simulink model "simCRM_Hybrid"  (R2016b)
settings: Solver=ode5  StartTime=0.0  StopTime=SimConfig.EndTime  FixedStep=SimConfig.SampleTime  RelTol=1e-3
undefined symbols (not defined in the file): CRM, WindReconstruction
libraries: lib_Sim_CRM x9, Controllers x1, Lidar_WindReconstruction x1, simulink x1
settings Model: Creator=cava_da  LastModifiedBy=cava_da
settings DataIOCC: Decimation=SimConfig.Logging.DecimationFactor  SaveFormat=StructureWithTime  ReturnWorkspaceOutputs=on
settings OptimizationCC: ExpressionDepthLimit=2147483647  InitFltsAndDblsToZero=on  LifeSpan=inf
settings DebuggingCC: UnderspecifiedInitializationDetection=Classic  MergeDetectMultiDrivingBlocksExec=none  SolverPrmCheckMsg=warning  FcnCallInpInsideContextMsg=warning  StateNameClashWarn=warning  SFUnexpectedBacktrackingDiag=warning  SFNoUnconditionalDefaultTransitionDiag=warning  SFExecutionAtInitializationDiag=none
settings HardwareCC: ProdBitPerPointer=32  ProdBitPerSizeT=32  ProdBitPerPtrDiffT=32  ProdLargestAtomicFloat=None  ProdIntDivRoundTo=Undefined  ProdEndianess=Unspecified  ProdWordSize=32  ProdHWDeviceType=32-bit Generic
settings ModelReferenceCC: PropagateSignalLabelsOutOfModel=off
settings SFSimCC: SimUseLocalCustomCode=on
settings RTWCC: RTWUseLocalCustomCode=on
settings GRTTargetCC: TargetLangStandard=C89/C90 (ANSI)  CombineOutputUpdateFcns=off  GRTInterface=on
settings ConfigComp: CovMetricSettings=dw  CovHtmlReporting=on  CovSaveCumulativeToWorkspaceVar=on  CovSaveSingleToWorkspaceVar=on

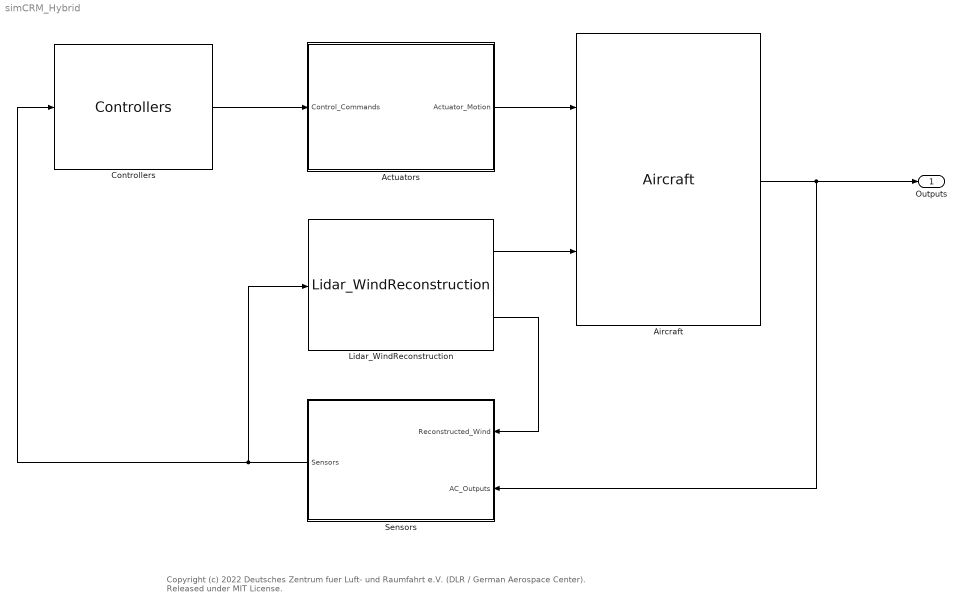
== system simCRM_Hybrid ==
  note: Copyright (c) 2022 Deutsches Zentrum fuer Luft- und Raumfahrt e.V. (DLR / German Aerospace Center). Released under MIT License.
  Actuators : Subsystem
  Aircraft : lib_Sim_CRM/Aircraft  modelName=CRM.Aircraft
  Controllers : Controllers/Controllers  SystemSampleTime=-1
  Lidar_WindReconstruction : Lidar_WindReconstruction/Lidar_WindReconstruction  SystemSampleTime=-1
  Sensors : Subsystem
  Outputs : Outport
  wires:
  Lidar_WindReconstruction/1 -> Aircraft/2
  Aircraft/1 -> Outputs/1, Sensors/2(AC_Outputs)
  Lidar_WindReconstruction/2 -> Sensors/1(Reconstructed_Wind)
  Sensors/1(Sensors) -> Controllers/1, Lidar_WindReconstruction/1
  Controllers/1 -> Actuators/1(Control_Commands)
  Actuators/1(Actuator_Motion) -> Aircraft/1

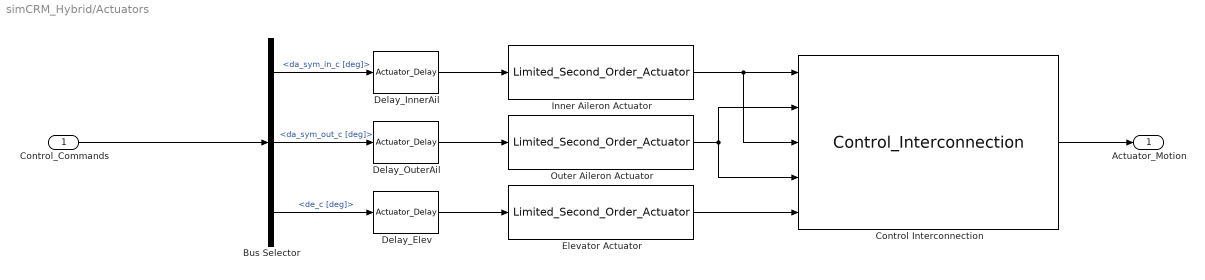
== system simCRM_Hybrid/Actuators ==
  Control_Commands : Inport
  Bus Selector : BusSelector  OutputSignals=da_sym_in_c [deg],da_sym_out_c [deg],de_c [deg]
  Control Interconnection : lib_Sim_CRM/Control_Interconnection
  Delay_Elev : lib_Sim_CRM/Actuator_Delay  Act_Delay=CRM.Actuators.Global_Delay
  Delay_InnerAil : lib_Sim_CRM/Actuator_Delay  Act_Delay=CRM.Actuators.Global_Delay
  Delay_OuterAil : lib_Sim_CRM/Actuator_Delay  Act_Delay=CRM.Actuators.Global_Delay
  Elevator Actuator : lib_Sim_CRM/Limited_Second_Order_Actuator  actuatorName=CRM.Actuators.Elevator
  Inner Aileron Actuator : lib_Sim_CRM/Limited_Second_Order_Actuator  actuatorName=CRM.Actuators.InnerAileron
  Outer Aileron Actuator : lib_Sim_CRM/Limited_Second_Order_Actuator  actuatorName=CRM.Actuators.OuterAileron
  Actuator_Motion : Outport
  wires:
  Inner Aileron Actuator/1 -> Control Interconnection/1, Control Interconnection/3
  Outer Aileron Actuator/1 -> Control Interconnection/4, Control Interconnection/2
  Elevator Actuator/1 -> Control Interconnection/5
  Bus Selector/1 -> Delay_InnerAil/1  "<da_sym_in_c [deg]>"
  Control Interconnection/1 -> Actuator_Motion/1
  Bus Selector/3 -> Delay_Elev/1  "<de_c [deg]>"
  Bus Selector/2 -> Delay_OuterAil/1  "<da_sym_out_c [deg]>"
  Control_Commands/1 -> Bus Selector/1
  Delay_Elev/1 -> Elevator Actuator/1
  Delay_InnerAil/1 -> Inner Aileron Actuator/1
  Delay_OuterAil/1 -> Outer Aileron Actuator/1

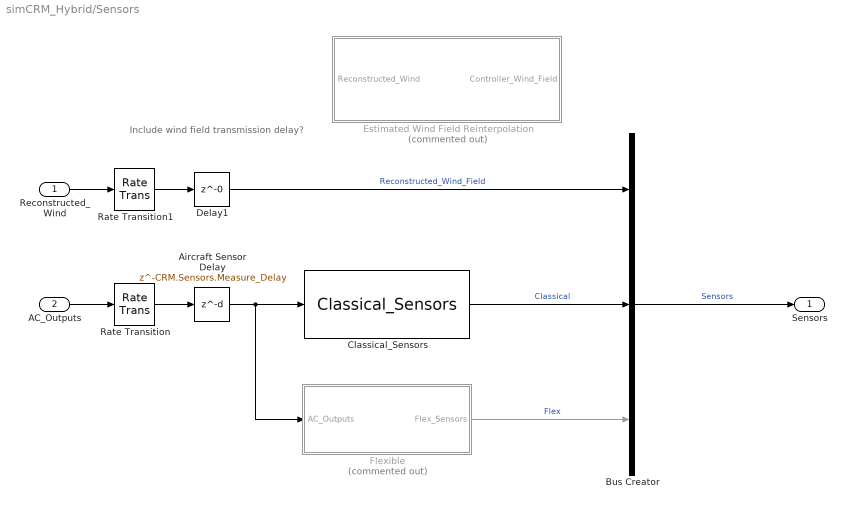
== system simCRM_Hybrid/Sensors ==
  note: Include wind field transmission delay?
  Reconstructed_Wind : Inport
  AC_Outputs : Inport  Port=2
  Aircraft Sensor Delay : Delay  DelayLength=CRM.Sensors.Measure_Delay
  Bus Creator : BusCreator  Inputs=3
  Classical_Sensors : lib_Sim_CRM/Classical_Sensors  SystemSampleTime=-1
  Delay1 : Delay  DelayLength=0
  Estimated Wind Field Reinterpolation : Subsystem  Commented=on
  Flexible : Subsystem  Commented=on
  Rate Transition : RateTransition  OutPortSampleTime=CRM.FCS.SampleTime
  Rate Transition1 : RateTransition  OutPortSampleTime=CRM.FCS.SampleTime
  Sensors : Outport
  wires:
  Bus Creator/1 -> Sensors/1  "Sensors"
  AC_Outputs/1 -> Rate Transition/1
  Classical_Sensors/1 -> Bus Creator/2  "Classical"
  Flexible/1(Flex_Sensors) -> Bus Creator/3  "Flex"
  Reconstructed_Wind/1 -> Rate Transition1/1
  Delay1/1 -> Bus Creator/1  "Reconstructed_Wind_Field"
  Aircraft Sensor Delay/1 -> Classical_Sensors/1, Flexible/1(AC_Outputs)
  Rate Transition1/1 -> Delay1/1
  Rate Transition/1 -> Aircraft Sensor Delay/1

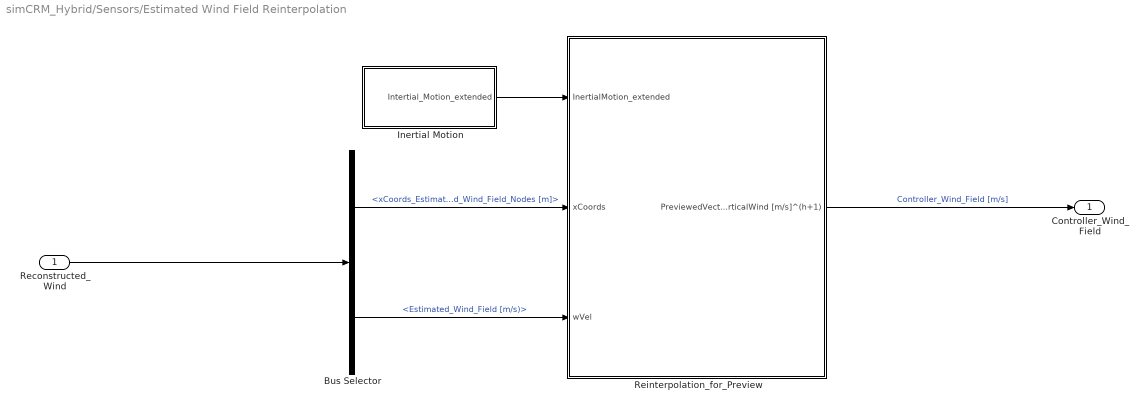
== system simCRM_Hybrid/Sensors/Estimated Wind Field Reinterpolation ==
  Reconstructed_Wind : Inport
  Bus Selector : BusSelector  OutputSignals=xCoords_Estimated_Wind_Field_Nodes [m],Estimated_Wind_Field [m/s)
  Inertial Motion : Subsystem
  Reinterpolation_for_Preview : Subsystem
  Controller_Wind_Field : Outport
  wires:
  Bus Selector/2 -> Reinterpolation_for_Preview/3(wVel)  "<Estimated_Wind_Field [m/s)>"
  Bus Selector/1 -> Reinterpolation_for_Preview/2(xCoords)  "<xCoords_Estimated_Wind_Field_Nodes [m]>"
  Reconstructed_Wind/1 -> Bus Selector/1
  Reinterpolation_for_Preview/1(PreviewedVectorOfVerticalWind [m/s]^(h+1)) -> Controller_Wind_Field/1  "Controller_Wind_Field [m/s]"
  Inertial Motion/1(Intertial_Motion_extended) -> Reinterpolation_for_Preview/1(InertialMotion_extended)

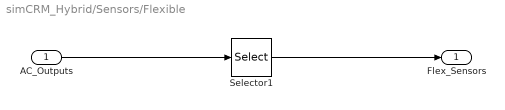
== system simCRM_Hybrid/Sensors/Flexible ==
  AC_Outputs : Inport
  Selector1 : Selector  InputPortWidth=25  IndexOptions=Index vector (dialog)  Indices=[1:25]  OutputSizes=1
  Flex_Sensors : Outport
  wires:
  AC_Outputs/1 -> Selector1/1
  Selector1/1 -> Flex_Sensors/1

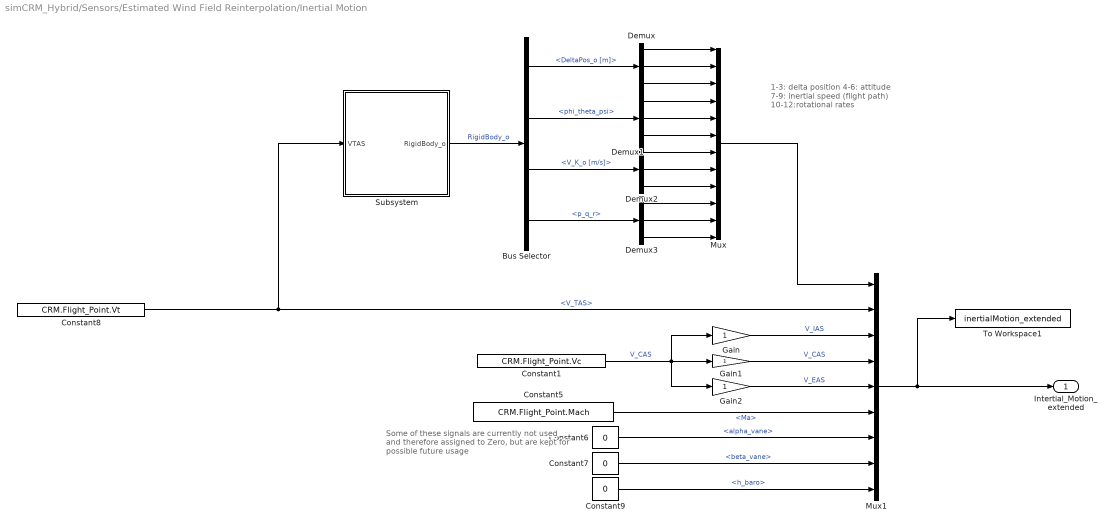
== system simCRM_Hybrid/Sensors/Estimated Wind Field Reinterpolation/Inertial Motion ==
  note: 1-3: delta position
      | 4-6: attitude
      | 7-9: inertial speed (flight path)
      | 10-12:rotational rates
  note: Some of these signals are currently not used
      |  and therefore assigned to Zero,
      | but are kept for possible future usage
  Bus Selector : BusSelector  OutputSignals=DeltaPos_o [m],phi_theta_psi,V_K_o [m/s],p_q_r
  Constant1 : Constant  Value=CRM.Flight_Point.Vc
  Constant5 : Constant  Value=CRM.Flight_Point.Mach
  Constant6 : Constant  Value=0
  Constant7 : Constant  Value=0
  Constant8 : Constant  Value=CRM.Flight_Point.Vt
  Constant9 : Constant  Value=0
  Demux{,1..3} (4 alike) : Demux  Outputs=3
  Gain : Gain
  Gain1 : Gain
  Gain2 : Gain
  Mux : Mux  Inputs=12
  Mux1 : Mux  Inputs=9
  Subsystem : Subsystem
  To Workspace1 : ToWorkspace  VariableName=inertialMotion_extended  SaveFormat=Structure  SampleTime=-1
  Intertial_Motion_extended : Outport
  wires:
  Bus Selector/4 -> Demux3/1  "<p_q_r>"
  Bus Selector/1 -> Demux/1  "<DeltaPos_o [m]>"
  Bus Selector/2 -> Demux1/1  "<phi_theta_psi>"
  Bus Selector/3 -> Demux2/1  "<V_K_o [m/s]>"
  Demux/1 -> Mux/1
  Demux/2 -> Mux/2
  Demux/3 -> Mux/3
  Demux1/1 -> Mux/4
  Demux1/2 -> Mux/5
  Demux1/3 -> Mux/6
  Demux2/1 -> Mux/7
  Demux2/2 -> Mux/8
  Demux2/3 -> Mux/9
  Demux3/1 -> Mux/10
  Demux3/2 -> Mux/11
  Demux3/3 -> Mux/12
  Mux1/1 -> Intertial_Motion_extended/1, To Workspace1/1
  Gain/1 -> Mux1/3  "V_IAS"
  Gain1/1 -> Mux1/4  "V_CAS"
  Gain2/1 -> Mux1/5  "V_EAS"
  Constant5/1 -> Mux1/6  "<Ma>"
  Constant6/1 -> Mux1/7  "<alpha_vane>"
  Constant7/1 -> Mux1/8  "<beta_vane>"
  Constant9/1 -> Mux1/9  "<h_baro>"
  Subsystem/1(RigidBody_o) -> Bus Selector/1  "RigidBody_o"
  Constant8/1 -> Subsystem/1(VTAS), Mux1/2  "<V_TAS>"
  Mux/1 -> Mux1/1
  Constant1/1 -> Gain2/1, Gain/1, Gain1/1  "V_CAS"

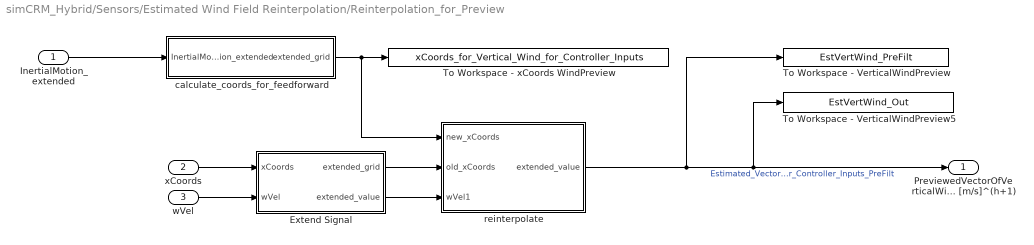
== system simCRM_Hybrid/Sensors/Estimated Wind Field Reinterpolation/Reinterpolation_for_Preview ==
  InertialMotion_extended : Inport
  xCoords : Inport  Port=2
  wVel : Inport  Port=3
  Extend Signal : Subsystem
  To Workspace - VerticalWindPreview : ToWorkspace  VariableName=EstVertWind_PreFilt  SampleTime=-1
  To Workspace - VerticalWindPreview5 : ToWorkspace  VariableName=EstVertWind_Out  SampleTime=-1
  To Workspace - xCoords WindPreview : ToWorkspace  VariableName=xCoords_for_Vertical_Wind_for_Controller_Inputs  SampleTime=-1
  calculate_coords_for_feedforward : Subsystem
  reinterpolate : Subsystem
  PreviewedVectorOfVerticalWind [m/s]^(h+1) : Outport
  wires:
  Extend Signal/2(extended_value) -> reinterpolate/3(wVel1)
  Extend Signal/1(extended_grid) -> reinterpolate/2(old_xCoords)
  reinterpolate/1(extended_value) -> PreviewedVectorOfVerticalWind [m/s]^(h+1)/1, To Workspace - VerticalWindPreview5/1, To Workspace - VerticalWindPreview/1  "Estimated_Vector_of_Vertical_Wind_for_Controller_Inputs_PreFilt"
  xCoords/1 -> Extend Signal/1(xCoords)
  wVel/1 -> Extend Signal/2(wVel)
  InertialMotion_extended/1 -> calculate_coords_for_feedforward/1(InertialMotion_extended)
  calculate_coords_for_feedforward/1(extended_grid) -> To Workspace - xCoords WindPreview/1, reinterpolate/1(new_xCoords)

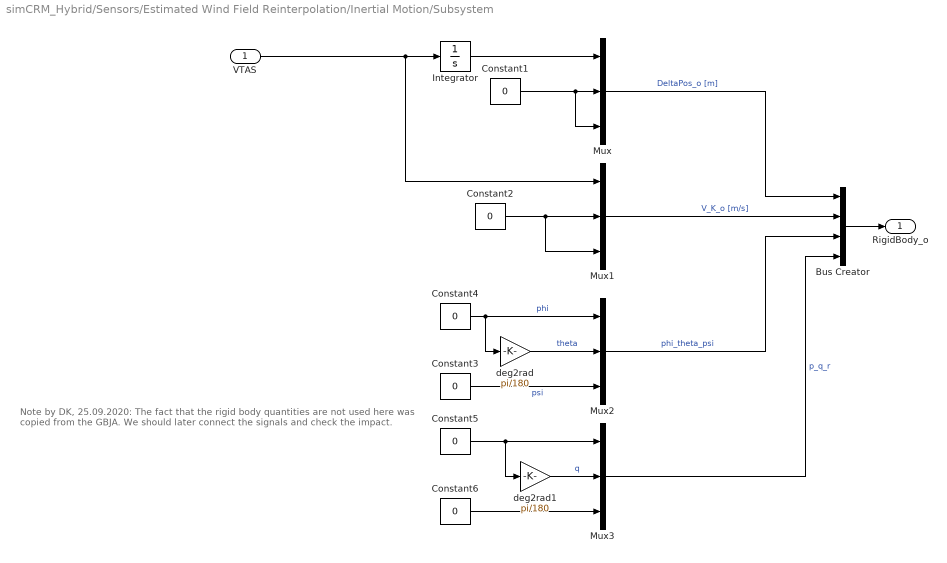
== system simCRM_Hybrid/Sensors/Estimated Wind Field Reinterpolation/Inertial Motion/Subsystem ==
  note: Note by DK, 25.09.2020:
      | The fact that the rigid body quantities are not used here was copied from the GBJA.
      | We should later connect the signals and check the impact.
  VTAS : Inport
  Bus Creator : BusCreator  Inputs=4
  Constant{1..6} (6 alike) : Constant  Value=0
  Integrator : Integrator
  Mux{,1..3} (4 alike) : Mux  Inputs=3
  deg2rad : Gain  Gain=pi/180
  deg2rad1 : Gain  Gain=pi/180
  RigidBody_o : Outport
  wires:
  Constant1/1 -> Mux/2, Mux/3
  Integrator/1 -> Mux/1
  Mux/1 -> Bus Creator/1  "DeltaPos_o [m]"
  Bus Creator/1 -> RigidBody_o/1
  Mux1/1 -> Bus Creator/2  "V_K_o [m/s]"
  Constant2/1 -> Mux1/2, Mux1/3
  Mux2/1 -> Bus Creator/3  "phi_theta_psi"
  Constant4/1 -> Mux2/1, deg2rad/1  "phi"
  deg2rad/1 -> Mux2/2  "theta"
  Constant3/1 -> Mux2/3  "psi"
  Mux3/1 -> Bus Creator/4  "p_q_r"
  deg2rad1/1 -> Mux3/2  "q"
  Constant5/1 -> Mux3/1, deg2rad1/1
  Constant6/1 -> Mux3/3
  VTAS/1 -> Mux1/1, Integrator/1

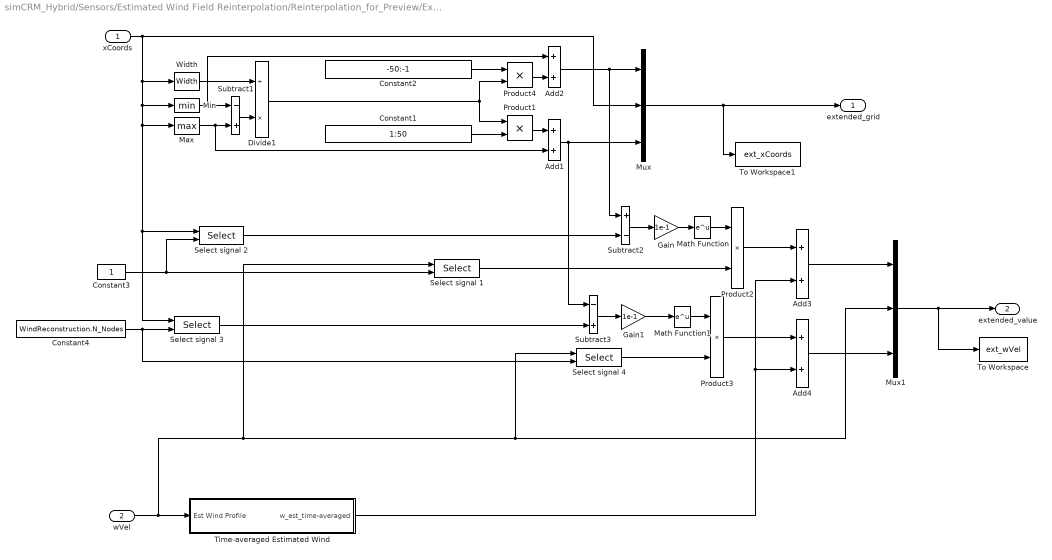
== system simCRM_Hybrid/Sensors/Estimated Wind Field Reinterpolation/Reinterpolation_for_Preview/Extend Signal ==
  xCoords : Inport
  wVel : Inport  Port=2
  Add{1..4} (4 alike) : Sum
  Constant1 : Constant  Value=1:50
  Constant2 : Constant  Value=-50:-1
  Constant3 : Constant
  Constant4 : Constant  Value=WindReconstruction.N_Nodes
  Divide1 : Product  Inputs=/*
  Gain : Gain  Gain=1e-1
  Gain1 : Gain  Gain=1e-1
  Math Function : Math  SaturateOnIntegerOverflow=on
  Math Function1 : Math  SaturateOnIntegerOverflow=on
  Max : MinMax  Function=max
  Min : MinMax
  Mux : Mux  Inputs=3
  Mux1 : Mux  Inputs=3
  Product{1..4} (4 alike) : Product  RndMeth=Zero
  Select signal {1..4} (4 alike) : Selector  InputPortWidth=WindReconstruction.N_Nodes  IndexOptions=Index vector (port)  Indices=1  OutputSizes=1
  Subtract1 : Sum  Inputs=-+
  Subtract2 : Sum  Inputs=+-
  Subtract3 : Sum  Inputs=-+
  Time-averaged Estimated Wind : Subsystem
  To Workspace : ToWorkspace  VariableName=ext_wVel  SaveFormat=Structure  SampleTime=-1
      settings: MaxDataPoints=100000
  To Workspace1 : ToWorkspace  VariableName=ext_xCoords  SaveFormat=Structure  SampleTime=-1
      settings: MaxDataPoints=100000
  Width : Width
  extended_grid : Outport
  extended_value : Outport  Port=2
  wires:
  xCoords/1 -> Min/1, Max/1, Select signal 2/1, Select signal 3/1, Width/1, Mux/2
  Time-averaged Estimated Wind/1(w_est_time-averaged) -> Add3/2, Add4/2
  wVel/1 -> Time-averaged Estimated Wind/1(Est Wind Profile), Select signal 1/1, Select signal 4/1, Mux1/2
  Max/1 -> Subtract1/2, Add1/2
  Subtract1/1 -> Divide1/2
  Width/1 -> Divide1/1
  Constant1/1 -> Product1/2
  Divide1/1 -> Product1/1, Product4/2
  Product1/1 -> Add1/1
  Min/1 -> Subtract1/1, Add2/1
  Product4/1 -> Add2/2
  Constant2/1 -> Product4/1
  Add1/1 -> Mux/3, Subtract3/1
  Add2/1 -> Mux/1, Subtract2/1
  Mux/1 -> extended_grid/1, To Workspace1/1
  Subtract2/1 -> Gain/1
  Math Function/1 -> Product2/1
  Select signal 1/1 -> Product2/2
  Product2/1 -> Add3/1
  Gain/1 -> Math Function/1
  Constant3/1 -> Select signal 1/2, Select signal 2/2
  Select signal 2/1 -> Subtract2/2
  Constant4/1 -> Select signal 3/2, Select signal 4/2
  Select signal 3/1 -> Subtract3/2
  Product3/1 -> Add4/1
  Math Function1/1 -> Product3/1
  Subtract3/1 -> Gain1/1
  Gain1/1 -> Math Function1/1
  Select signal 4/1 -> Product3/2
  Add3/1 -> Mux1/1
  Add4/1 -> Mux1/3
  Mux1/1 -> To Workspace/1, extended_value/1

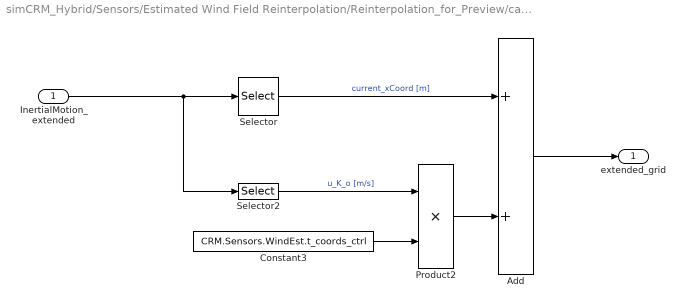
== system simCRM_Hybrid/Sensors/Estimated Wind Field Reinterpolation/Reinterpolation_for_Preview/calculate_coords_for_feedforward ==
  InertialMotion_extended : Inport
  Add : Sum
  Constant3 : Constant  Value=CRM.Sensors.WindEst.t_coords_ctrl
  Product2 : Product  RndMeth=Zero
  Selector : Selector  InputPortWidth=20  IndexOptions=Index vector (dialog)  Indices=1  OutputSizes=1
  Selector2 : Selector  InputPortWidth=20  IndexOptions=Index vector (dialog)  Indices=7  OutputSizes=1
  extended_grid : Outport
  wires:
  InertialMotion_extended/1 -> Selector2/1, Selector/1
  Selector/1 -> Add/1  "current_xCoord [m]"
  Product2/1 -> Add/2
  Add/1 -> extended_grid/1
  Selector2/1 -> Product2/1  "u_K_o [m/s]"
  Constant3/1 -> Product2/2

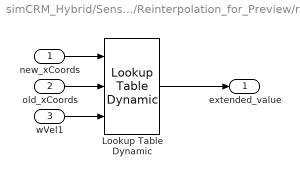
== system simCRM_Hybrid/Sensors/Estimated Wind Field Reinterpolation/Reinterpolation_for_Preview/reinterpolate ==
  new_xCoords : Inport
  old_xCoords : Inport  Port=2
  wVel1 : Inport  Port=3
  Lookup Table Dynamic : simulink/Lookup Tables/Lookup Table Dynamic  LookUpMeth=Interpolation-Use End Values  OutDataType=float('double')  OutScaling=[]  OutputDataTypeScalingMode=Specify via dialog  OutDataTypeStr=float('double')  DoSatur=off
  extended_value : Outport
  wires:
  old_xCoords/1 -> Lookup Table Dynamic/2
  wVel1/1 -> Lookup Table Dynamic/3
  Lookup Table Dynamic/1 -> extended_value/1
  new_xCoords/1 -> Lookup Table Dynamic/1

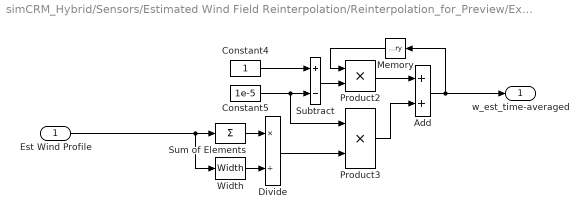
== system simCRM_Hybrid/Sensors/Estimated Wind Field Reinterpolation/Reinterpolation_for_Preview/Extend Signal/Time-averaged Estimated Wind ==
  Est Wind Profile : Inport
  Add : Sum
  Constant4 : Constant
  Constant5 : Constant  Value=1e-5
  Divide : Product  Inputs=*/
  Memory : Memory
  Product2 : Product  RndMeth=Zero
  Product3 : Product  RndMeth=Zero
  Subtract : Sum  Inputs=+-
  Sum of Elements : Sum  Inputs=+
  Width : Width
  w_est_time-averaged : Outport
  wires:
  Sum of Elements/1 -> Divide/1
  Width/1 -> Divide/2
  Constant4/1 -> Subtract/1
  Constant5/1 -> Subtract/2, Product3/1
  Add/1 -> Memory/1, w_est_time-averaged/1
  Product2/1 -> Add/1
  Subtract/1 -> Product2/2
  Memory/1 -> Product2/1
  Product3/1 -> Add/2
  Divide/1 -> Product3/2
  Est Wind Profile/1 -> Sum of Elements/1, Width/1
